simulink model "T1_simulink"  (R2024b)
settings: Solver=VariableStepAuto  StartTime=0.0  StopTime=30  RelTol=1e-3
libraries: simulink x1
settings Model: Creator=LUCAS  LastModifiedBy=gmspe
settings RTWCC: GPUComputeCapability=3.5

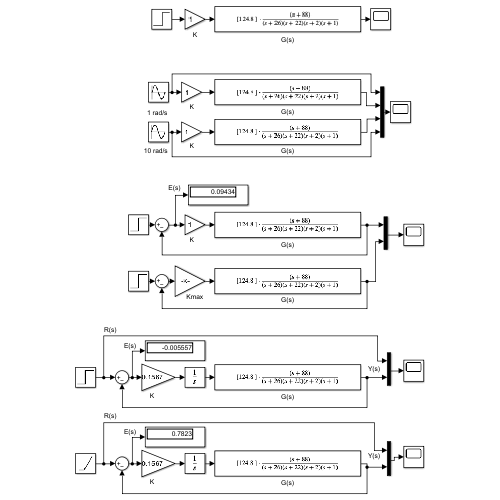
[thumbnail: Simulink's stored preview of the top-level diagram]
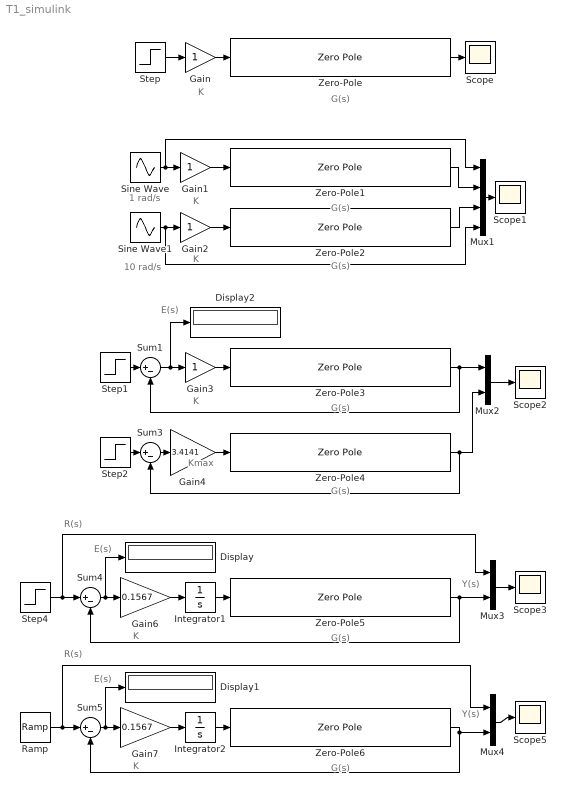
== system T1_simulink ==
  note: Kmax
  note: K
  note: G(s)
  note: K
  note: G(s)
  note: K
  note: G(s)
  note: 1 rad/s
  note: 10 rad/s
  note: G(s)
  note: K
  note: G(s)
  note: K
  note: G(s)
  note: E(s)
  note: R(s)
  note: E(s)
  note: G(s)
  note: R(s)
  note: K
  note: Y(s)
  note: Y(s)
  note: E(s)
  Display : Display
  Display1 : Display
  Display2 : Display
  Gain{,1..3} (4 alike) : Gain
  Gain4 : Gain  Gain=3.4141
  Gain6 : Gain  Gain=0.1567
  Gain7 : Gain  Gain=0.1567
  Integrator1 : Integrator
  Integrator2 : Integrator
  Mux1 : Mux
  Mux2 : Mux  Inputs=2
  Mux3 : Mux  Inputs=2
  Mux4 : Mux  Inputs=2
  Ramp : simulink/Sources/Ramp  slope=1  start=0  InitialOutput=0
  Scope{,1..3,5} (5 alike) : Scope
  Sine Wave : Sin  SampleTime=0
  Sine Wave1 : Sin  Frequency=10  SampleTime=0
  Step{,1..2,4} (4 alike) : Step  SampleTime=0
  Sum{1,3..5} (4 alike) : Sum  Inputs=|+-
  Zero-Pole{,1..6} (7 alike) : ZeroPole  Zeros=[-88]  Poles=[-26 -22 -2 -1]  Gain=[124.8]
  wires:
  Step/1 -> Gain/1
  Gain/1 -> Zero-Pole/1
  Zero-Pole/1 -> Scope/1
  Sine Wave/1 -> Mux1/1, Gain1/1
  Gain1/1 -> Zero-Pole1/1
  Mux1/1 -> Scope1/1
  Zero-Pole1/1 -> Mux1/2
  Zero-Pole2/1 -> Mux1/3
  Sine Wave1/1 -> Mux1/4, Gain2/1
  Gain2/1 -> Zero-Pole2/1
  Mux2/1 -> Scope2/1
  Gain4/1 -> Zero-Pole4/1
  Zero-Pole4/1 -> Sum3/2, Mux2/2
  Gain3/1 -> Zero-Pole3/1
  Zero-Pole3/1 -> Sum1/2, Mux2/1
  Step1/1 -> Sum1/1
  Step2/1 -> Sum3/1
  Sum3/1 -> Gain4/1
  Step4/1 -> Mux3/1, Sum4/1
  Sum4/1 -> Display/1, Gain6/1
  Zero-Pole5/1 -> Mux3/2, Sum4/2
  Mux3/1 -> Scope3/1
  Integrator1/1 -> Zero-Pole5/1
  Gain6/1 -> Integrator1/1
  Gain7/1 -> Integrator2/1
  Zero-Pole6/1 -> Mux4/2, Sum5/2
  Sum5/1 -> Display1/1, Gain7/1
  Mux4/1 -> Scope5/1
  Ramp/1 -> Mux4/1, Sum5/1
  Integrator2/1 -> Zero-Pole6/1
  Sum1/1 -> Display2/1, Gain3/1
